simulink model "TUNNINGPID"  (R2023b)
settings: Solver=VariableStepAuto  StartTime=0.0  StopTime=200  RelTol=1e-3
model workspace (MAT data in the model file):
  DOWN_TABLE = Simulink.Parameter
  DOWN_TABLE.Value = [0  5  28.5  40  64.8; 0  5  28.5  41.9  55.7; 0  5  28.5  50  68.7; 0  5.2  34.9  61.5  78.7; 0  15.3  40.1  64.1  82.1; 0  25.4  45.1  68.7  87.7; 0  30  47.5  70  89]
  DOWN_TABLE.DataType = 'auto'
  DOWN_TABLE.Complexity = 'real'
  DOWN_TABLE.Dimensions = [7 5]
  DOWN_TH_BP = Simulink.Parameter
  DOWN_TH_BP.Value = [0; 0.15; 0.33; 0.5; 0.67; 0.83; 1]
  DOWN_TH_BP.DataType = 'auto'
  DOWN_TH_BP.Complexity = 'real'
  DOWN_TH_BP.Dimensions = [7 1]
  TWAIT = Simulink.Parameter
  TWAIT.Value = 2
  TWAIT.DataType = 'auto'
  TWAIT.Complexity = 'real'
  TWAIT.Dimensions = [1 1]
  UP_TABLE = Simulink.Parameter
  UP_TABLE.Value = [10  31.4  50  70  1000000; 10.1  32  51.5  70.4  1000000; 13.2  37  61  72  1000000; 18.4  44  70  84.9  1000000; 24.8  48  74  88.7  1000000; 31  51.2  78  94.5  100000; 33.2  52.5  80  89  100000]
  UP_TABLE.DataType = 'auto'
  UP_TABLE.Complexity = 'real'
  UP_TABLE.Dimensions = [7 5]
  UP_TH_BP = Simulink.Parameter
  UP_TH_BP.Value = [0; 0.15; 0.33; 0.5; 0.67; 0.83; 1]
  UP_TH_BP.DataType = 'auto'
  UP_TH_BP.Complexity = 'real'
  UP_TH_BP.Dimensions = [7 1]
libraries: slpidlib x1
settings Model: Creator=Admin  LastModifiedBy=Admin

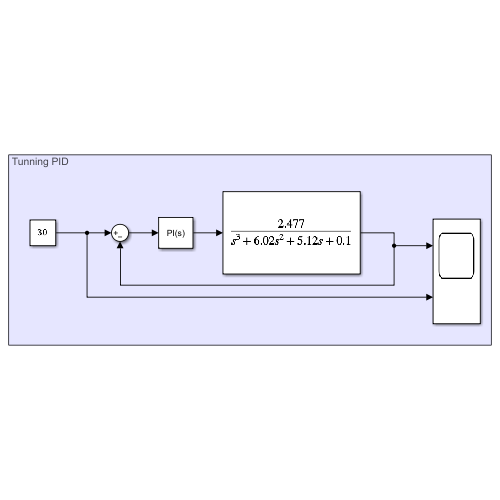
[thumbnail: Simulink's stored preview of the top-level diagram]
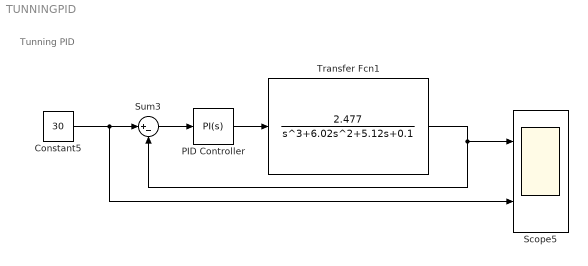
== system TUNNINGPID ==
  note: Tunning PID
  Constant5 : Constant  Value=30
  PID Controller : slpidlib/PID Controller  Controller=PI  Form=Parallel  TimeDomain=Continuous-time  UseExternalTs=off  SampleTime=-1  IntegratorMethod=Forward Euler  FilterMethod=Forward Euler  ControllerParametersSource=internal  P=0.470258928206213  I=0.0109019601067834  UseKiTs=off  D=8.181378548763  N=350  UseFilter=on  TunerSelectOption=Transfer Function Based (PID Tuner App)  InitialConditionSource=internal  InitialConditionForIntegrator=0  InitialConditionForFilter=0  DifferentiatorICPrevScaledInput=0  ExternalReset=none  TrackingMode=off  Kt=1  LimitOutput=off  SatLimitsSource=internal  UpperSaturationLimit=1  LowerSaturationLimit=-1  LinearizeAsGain=on  AntiWindupMode=none  Kb=1  LimitIntegrator=off  UpperIntegratorSaturationLimit=inf  LowerIntegratorSaturationLimit=-inf  POutMin=[]  POutMax=[]  IOutMin=[]  IOutMax=[]  DOutMin=[]  DOutMax=[]  NOutMin=[]  NOutMax=[]  SumOutMin=[]  SumOutMax=[]  SaturationOutMin=[]  SaturationOutMax=[]  PParamMin=[]  PParamMax=[]  IParamMin=[]  IParamMax=[]  DParamMin=[]  DParamMax=[]  NParamMin=[]  NParamMax=[]  KbParamMin=[]  KbParamMax=[]  KtParamMin=[]  KtParamMax=[]  KbOutMin=[]  KbOutMax=[]  KtOutMin=[]  KtOutMax=[]  IntegratorOutMin=[]  IntegratorOutMax=[]  FilterOutMin=[]  FilterOutMax=[]  SumI1OutMin=[]  SumI1OutMax=[]  SumI2OutMin=[]  SumI2OutMax=[]  SumI3OutMin=[]  SumI3OutMax=[]  SumI4OutMin=[]  SumI4OutMax=[]  SumDOutMin=[]  SumDOutMax=[]  DifferentiatorOutMin=[]  DifferentiatorOutMax=[]  FilterDiffOutCoefMin=[]  FilterDiffOutCoefMax=[]  ReciprocalOutMin=[]  ReciprocalOutMax=[]  SumDenOutMin=[]  SumDenOutMax=[]  SumNumOutMin=[]  SumNumOutMax=[]  DivideOutMin=[]  DivideOutMax=[]  UdiffTsProdOutMin=[]  UdiffTsProdOutMax=[]  NTsProdOutMin=[]  NTsProdOutMax=[]  UintegralTsProdOutMin=[]  UintegralTsProdOutMax=[]  UngainTsProdOutMin=[]  UngainTsProdOutMax=[]  ClampingZeroOutDataTypeStr=Inherit: Inherit via back propagation  ClampingZeroOutMin=[]  ClampingZeroOutMax=[]  FilterDenConstantOutDataTypeStr=Inherit: Inherit via back propagation  FilterDenConstantOutMin=[]  FilterDenConstantOutMax=[]  PCopyOutDataTypeStr=Inherit: Inherit via back propagation  PCopyOutMin=[]  PCopyOutMax=[]  NCopyOutDataTypeStr=Inherit: Inherit via back propagation  NCopyOutMin=[]  NCopyOutMax=[]  IntegratorContinuousStateAttributes=''  IntegratorStateMustResolveToSignalObject=off  IntegratorRTWStateStorageClass=Auto  FilterContinuousStateAttributes=''  FilterStateMustResolveToSignalObject=off  FilterRTWStateStorageClass=Auto  ParallelPVariant=InternalParameters  IdealPVariant=Disabled  IVariant=InternalParameters  DVariant=Disabled  IntegratorVariant=Continuous  SatVariant=Disabled  AWVariant=Passthrough  PCopyVariant=Disabled  TRVariant=Disabled  FdbkBlocksVariant=Forward  IdealPFdbkVariant=Disabled  SatFdbkVariant=Disabled  DerivativeFilterVariant=Disabled  NVariant=Disabled  NCopyVariant=Disabled_SignalSpec  FilterICVariant=Disabled  IntegratorICVariant=InternalICs  ExternalResetVariant=Disabled  TRSumVariant=Passthrough  SumFdbkVariant=Disabled  SumVariant=Sum_PI  TsampFilterVariant=InternalTs  TsampNgainVariant=Passthrough  TsampIntegralVariant=Disabled_SignalSpec  ExternalSaturationOutDataTypeStr=Inherit: Same as second input
  Scope5 : Scope  NumInputPorts=2
  Sum3 : Sum  Inputs=|+-
  Transfer Fcn1 : TransferFcn  Numerator=[2.477]  Denominator=[1 6.02 5.12 0.1]
  wires:
  Constant5/1 -> Scope5/2, Sum3/1
  Sum3/1 -> PID Controller/1
  PID Controller/1 -> Transfer Fcn1/1
  Transfer Fcn1/1 -> Sum3/2, Scope5/1
